simulink library "Driver_Override_None"  (R2025b)
settings: Solver=VariableStepAuto  StartTime=0.0  StopTime=10.0  RelTol=1e-3
undefined symbols (not defined in the file): Scene
Description:
  | Simscape Vehicle Templates Library
  | 
  | Copyright 2018-2025 The MathWorks, Inc.
settings Model: Creator=smiller  LastModifiedBy=smiller
settings OptimizationCC: ReuseModelBlockBuffer=off
settings ModelReferenceCC: EnableRefExpFcnMdlSchedulingChecks=on
settings RTWCC: GPUComputeCapability=3.5

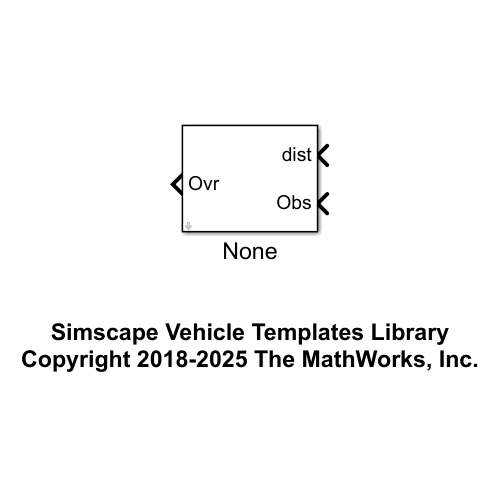
[thumbnail: Simulink's stored preview of the top-level diagram]
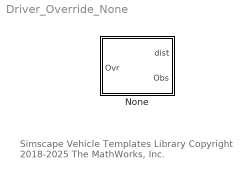
== system Driver_Override_None ==
  note: Simscape Vehicle Templates Library
      | Copyright 2018-2025 The MathWorks, Inc.
  None : Subsystem  VariantControl=None  mask(No Driver Override){override=Scene.Mallory_Park_Obstacle.Override}
      mask prompts: override "Override parameters (structure)"
      mask help: Driver commands are not overridden, regardless of inputs to subsystem.

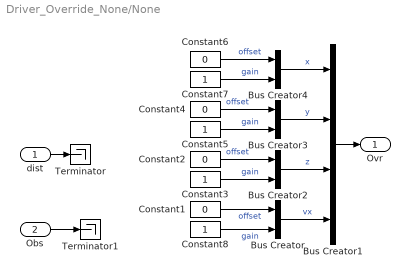
== system Driver_Override_None/None ==
  dist : Inport
  Obs : Inport  Port=2
  Bus Creator{,2..4} (4 alike) : BusCreator  Inputs=2
  Bus Creator1 : BusCreator  Inputs=4
  Constant{1..2,4,6} (4 alike) : Constant  Value=0
  Constant{3,5,7..8} (4 alike) : Constant
  Terminator : Terminator
  Terminator1 : Terminator
  Ovr : Outport  VectorParamsAs1DForOutWhenUnconnected=off
  wires:
  dist/1 -> Terminator/1
  Obs/1 -> Terminator1/1
  Bus Creator1/1 -> Ovr/1
  Constant1/1 -> Bus Creator/1  "offset"
  Constant8/1 -> Bus Creator/2  "gain"
  Constant6/1 -> Bus Creator4/1  "offset"
  Constant7/1 -> Bus Creator4/2  "gain"
  Constant5/1 -> Bus Creator3/2  "gain"
  Constant4/1 -> Bus Creator3/1  "offset"
  Constant3/1 -> Bus Creator2/2  "gain"
  Bus Creator2/1 -> Bus Creator1/3  "z"
  Constant2/1 -> Bus Creator2/1  "offset"
  Bus Creator3/1 -> Bus Creator1/2  "y"
  Bus Creator/1 -> Bus Creator1/4  "vx"
  Bus Creator4/1 -> Bus Creator1/1  "x"
